simulink model "pruebarc"  (R2025a)
settings: Solver=FixedStepAuto  StartTime=0.0  StopTime=inf  FixedStep=0.001  RelTol=1e-3  EnableMultiTasking=on
model workspace (MAT data in the model file):
  F = [-0.7032  -0.5711  1.7669; 0.2778  -1.4711  1.3647; -0.2558  -0.048  -0.058; -0.11613436  1.15693153  -2.12434445; -0.9531108  1.93997803  -1.59591795; 0.18138056  0.21948418  -0.51411462; 0.946468571296  -1.53366910719  1.49687863641; 1.6173892229  -2.23297604045  1.05599978612; 0.064936415208  -0.401792113254  0.64983001987; -1.4745115325  1.64380224797  -0.507501872867; -2.02779359087  2.31055207818  -0.250825372052; -0.323507655319  0.522799350129  -0.471279686079; 1.62334375322  -1.55174386087  -0.332582390354; 2.13197695059  -2.2289406246  -0.415150203049; 0.493277586385  -0.56171347709  0.16919281873]
  G = [4.2242  -1.1144  -1.3646  0  0  0  0  0  0  0  0  0  0  0  0; -0.011  -5.2505  -0.6752  0  0  0  0  0  0  0  0  0  0  0  0; 0.4464  -0.0899  0.7457  0  0  0  0  0  0  0  0  0  0  0  0; -2.17543118  3.62336232  2.66277077  4.2242  -1.1144  -1.3646  0  0  0  0  0  0  0  0  0; 1.79886694  7.2917437  1.63185763  -0.011  -5.2505  -0.6752  0  0  0  0  0  0  0  0  0; -1.10591356  0.54230172  0.33822368  0.4464  -0.0899  0.7457  0  0  0  0  0  0  0  0  0; -1.45160837282  -5.75407030143  -2.20680687777  -2.17543118  3.62336232  2.66277077  4.2242  -1.1144  -1.3646  0  0  0  0  0  0; -4.75988817257  -8.98023494729  -1.19933418349  1.79886694  7.2917437  1.63185763  -0.011  -5.2505  -0.6752  0  0  0  0  0  0; 0.534272669204  -1.30831327882  -0.779082902646  -1.10591356  0.54230172  0.33822368  0.4464  -0.0899  0.7457  0  0  0  0  0  0; 4.68314952234  6.86321568202  0.860204767951  -1.45160837282  -5.75407030143  -2.20680687777  -2.17543118  3.62336232  2.66277077  4.2242  -1.1144  -1.3646  0  0  0; 7.32813659636  9.82688776962  0.0880751294495  -4.75988817257  -8.98023494729  -1.19933418349  1.79886694  7.2917437  1.63185763  -0.011  -5.2505  -0.6752  0  0  0; 0.568808239237  1.97882463075  0.667256048493  0.534272669204  -1.30831327882  -0.779082902646  -1.10591356  0.54230172  0.33822368  0.4464  -0.0899  0.7457  0  0  0; -6.47326227638  -6.94196363276  0.523779012831  4.68314952234  6.86321568202  0.860204767951  -1.45160837282  -5.75407030143  -2.20680687777  -2.17543118  3.62336232  2.66277077  4.2242  -1.1144  -1.3646; -8.70319020551  -9.84923130785  1.02000189098  7.32813659636  9.82688776962  0.0880751294495  -4.75988817257  -8.98023494729  -1.19933418349  1.79886694  7.2917437  1.63185763  -0.011  -5.2505  -0.6752; -1.58269108232  -2.34207301299  -0.262968836668  0.568808239237  1.97882463075  0.667256048493  0.534272669204  -1.30831327882  -0.779082902646  -1.10591356  0.54230172  0.33822368  0.4464  -0.0899  0.7457]
  H = [22131.1173138 20323.7560581 -1531.64777338 -13284.6672436 -19882.239349 -1189.60000517 7040.1548235 16995.1890063 2962.85657152 -1788.53809124 -12245.5245907 -3182.80208225 ... (225 elements, 15x15)]
  Pc = [-4.2242 0.011 -0.4464 4.2242 -0.011 0.4464 2.17543118 -1.79886694 1.10591356 -2.17543118 1.79886694 -1.10591356 ... (1020 elements, 68x15)]
  Qvec = [50  0  0  0  0  0  0  0  0  0  0  0  0  0  0; 0  50  0  0  0  0  0  0  0  0  0  0  0  0  0; 0  0  50  0  0  0  0  0  0  0  0  0  0  0  0; 0  0  0  50  0  0  0  0  0  0  0  0  0  0  0; 0  0  0  0  50  0  0  0  0  0  0  0  0  0  0; 0  0  0  0  0  50  0  0  0  0  0  0  0  0  0; 0  0  0  0  0  0  50  0  0  0  0  0  0  0  0; 0  0  0  0  0  0  0  50  0  0  0  0  0  0  0; 0  0  0  0  0  0  0  0  50  0  0  0  0  0  0; 0  0  0  0  0  0  0  0  0  50  0  0  0  0  0; 0  0  0  0  0  0  0  0  0  0  50  0  0  0  0; 0  0  0  0  0  0  0  0  0  0  0  50  0  0  0; 0  0  0  0  0  0  0  0  0  0  0  0  122.671454978  -50.1228812954  -14.951064512; 0  0  0  0  0  0  0  0  0  0  0  0  -50.1228812954  218.216126937  -177.895514013; 0  0  0  0  0  0  0  0  0  0  0  0  -14.951064512  -177.895514013  361.167619907]
  Sc = [-0.7032  -0.5711  1.7669; 0.2778  -1.4711  1.3647; -0.2558  -0.048  -0.058; 0.7032  0.5711  -1.7669; -0.2778  1.4711  -1.3647; 0.2558  0.048  0.058; -0.11613436  1.15693153  -2.12434445; -0.9531108  1.93997803  -1.59591795; 0.18138056  0.21948418  -0.51411462; 0.11613436  -1.15693153  2.12434445; 0.9531108  -1.93997803  1.59591795; -0.18138056  -0.21948418  0.51411462; 0.946468571296  -1.53366910719  1.49687863641; 1.6173892229  -2.23297604045  1.05599978612; 0.064936415208  -0.401792113254  0.64983001987; -0.946468571296  1.53366910719  -1.49687863641; -1.6173892229  2.23297604045  -1.05599978612; -0.064936415208  0.401792113254  -0.64983001987; -1.4745115325  1.64380224797  -0.507501872867; -2.02779359087  2.31055207818  -0.250825372052; -0.323507655319  0.522799350129  -0.471279686079; 1.4745115325  -1.64380224797  0.507501872867; 2.02779359087  -2.31055207818  0.250825372052; 0.323507655319  -0.522799350129  0.471279686079; 1.62334375322  -1.55174386087  -0.332582390354; 2.13197695059  -2.2289406246  -0.415150203049; 0.493277586385  -0.56171347709  0.16919281873; -1.62334375322  1.55174386087  0.332582390354; -2.13197695059  2.2289406246  0.415150203049; -0.493277586385  0.56171347709  -0.16919281873; 0  0  0; 0  0  0; 0  0  0; 0  0  0; 0  0  0; 0  0  0; 0  0  0; 0  0  0; 0  0  0; 0  0  0; 0  0  0; 0  0  0; 0  0  0; 0  0  0; 0  0  0; 0  0  0; 0  0  0; 0  0  0; 0  0  0; 0  0  0; 0  0  0; 0  0  0; 0  0  0; 0  0  0; 0  0  0; 0  0  0; 0  0  0; 0  0  0; 0  0  0; 0  0  0; -1.01143611879  0.934917795451  0.497586139165; 1.01143611879  -0.934917795451  -0.497586139165; 1.62334375322  -1.55174386087  -0.332582390354; 2.13197695059  -2.2289406246  -0.415150203049; 0.493277586385  -0.56171347709  0.16919281873; -1.62334375322  1.55174386087  0.332582390354; -2.13197695059  2.2289406246  0.415150203049; -0.493277586385  0.56171347709  -0.16919281873]
  m = 3
  nu = 15
  qc = [1; 1; 0.5; 1; 1; 0.5; 1; 1; 0.5; 1; 1; 0.5; 1; 1; 0.5; 1; 1; 0.5; 1; 1; 0.5; 1; 1; 0.5; 1; 1; 0.5; 1; 1; 0.5; 1.41421356237; 1.41421356237; 2; 1.41421356237; 1.41421356237; 2; 1.41421356237; 1.41421356237; 2; 1.41421356237; 1.41421356237; 2; 1.41421356237; 1.41421356237; 2; 1.41421356237; 1.41421356237; 2; 1.41421356237; 1.41421356237; 2; 1.41421356237; 1.41421356237; 2; 1.41421356237; 1.41421356237; 2; 1.41421356237; 1.41421356237; 2; 1; 1; 1; 1; 0.5; 1; 1; 0.5]
libraries: px4Sensorslib x1
settings Model: SimulationMode=external  ExtModeTrigDuration=10  Creator=The MathWorks, Inc.  LastModifiedBy=aero
settings SolverCC: AlgebraicLoopSolver=TrustRegion  PositivePriorityOrder=on  AutoInsertRateTranBlk=on  MaxZcPerStep=1.0
settings OptimizationCC: EnhancedBackFolding=on  PassReuseOutputArgsAs=Individual arguments  MaxStackSize=64  OptimizeBlockOrder=speed  DifferentSizesBufferReuse=on  OptimizationCustomize=off  EfficientTunableParamExpr=on
settings DebuggingCC: ParameterPrecisionLossMsg=none  ParameterTunabilityLossMsg=error  UnconnectedInputMsg=warning  UnconnectedOutputMsg=warning  UnconnectedLineMsg=warning  SubsystemReferenceDiagnosticForUnitTest=warning  ArithmeticOperatorsInVariantConditions=warning
settings HardwareCC: ProdBitPerPointer=32.0  ProdBitPerSizeT=32.0  ProdBitPerPtrDiffT=32.0  ProdLargestAtomicInteger=Long  ProdLargestAtomicFloat=Double  ProdWordSize=32.0  ProdLongLongMode=on  ProdHWDeviceType=ARM Compatible->ARM Cortex
settings ModelReferenceCC: EnableRefExpFcnMdlSchedulingChecks=on
settings SFSimCC: MATLABDynamicMemAlloc=off  SimTargetLang=C++  SimDLTargetLibrary=mkl-dnn
settings RTWCC: SystemTargetFile=ert.tlc  HardwareBoard=PX4 Pixhawk 6c  TLCOptions="-aInlineSetEventsForThisBaseRateFcn=TLC_FALSE -aSuppressMultiTaskScheduler=TLC_FALSE  -aRateBasedStepFcn=0"  TemplateMakefile=ert_default_tmf  GenerateReport=on  Toolchain=GNU Tools for PX4 Autopilots  IncludeHyperlinkInReport=on  LaunchReport=on  TargetLang=C++  GenerateTraceInfo=on  GenerateTraceReport=on  GenerateTraceReportSl=on  GenerateTraceReportSf=on  GenerateTraceReportEml=on  GPUComputeCapability=3.5  DLArmComputeVersion=19.05  Description=Embedded Coder
settings CodeAppCC: ForceParamTrailComments=on  IgnoreCustomStorageClasses=off  OperatorAnnotations=on  SimulinkDataObjDesc=on  SFDataObjDesc=on  InsertBlockDesc=on
settings ERTTargetCC: ExtModeTransport=3.0  ExtModeStaticAllocSize=1024.0  InlinedParameterPlacement=Hierarchical

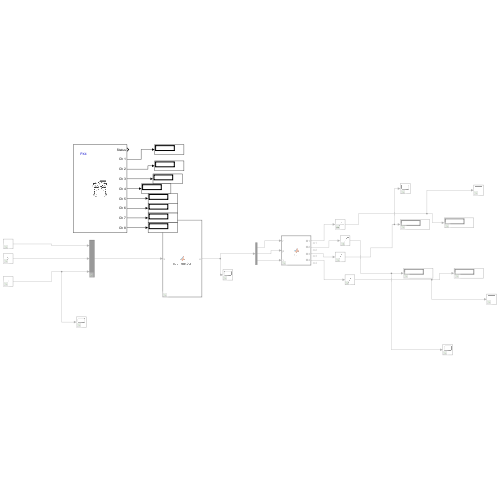
[thumbnail: Simulink's stored preview of the top-level diagram]
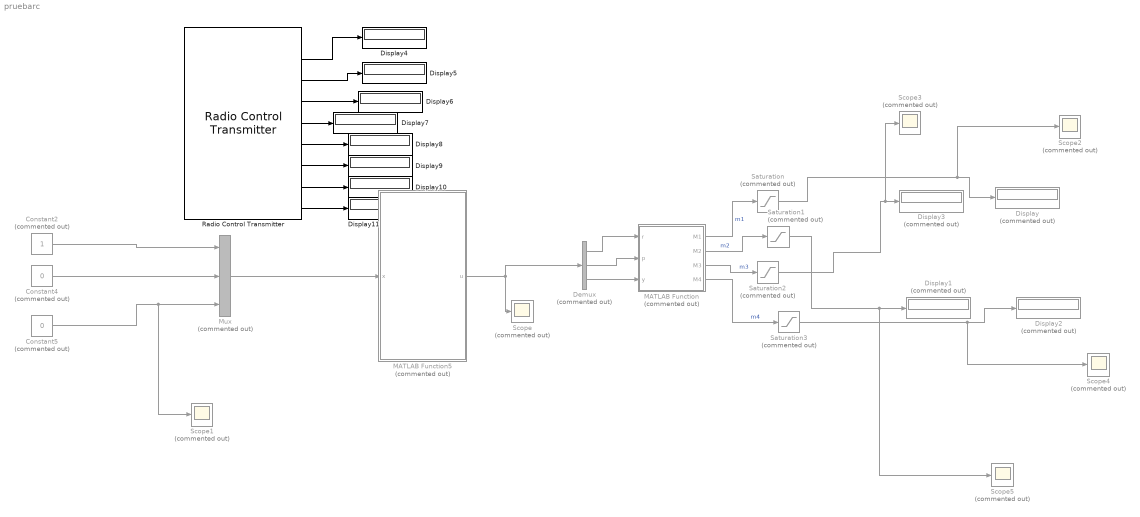
== system pruebarc ==
  Constant2 : Constant  Commented=on
  Constant4 : Constant  Commented=on  Value=0
  Constant5 : Constant  Commented=on  Value=0
  Demux : Demux  Commented=on  Outputs=3
  Display{,1..3} (4 alike) : Display  Commented=on
  Display{4..11} (8 alike) : Display
  MATLAB Function : MATLAB Function  Commented=on  TreatAsAtomicUnit=on  SystemSampleTime=0.0201
  MATLAB Function5 : MATLAB Function  Commented=on  TreatAsAtomicUnit=on  SystemSampleTime=0.0201
  Mux : Mux  Commented=on  Inputs=3
  Radio Control Transmitter : px4Sensorslib/Radio Control Transmitter  channel1=on  channel2=on  channel3=on  channel4=on  channel5=on  channel6=on  channel7=on  channel8=on  channel_count=off  rssi=off  rc_input_source=off  timestamp_last_signal=off  time_stamp=off  sampleTime=1/250  BlockingMode=off  BlockTimeout=5
  Saturation{,1..3} (4 alike) : Saturate  Commented=on  UpperLimit=1  LowerLimit=0
  Scope{,1..5} (6 alike) : Scope  Commented=on
      Scope settings: ActiveDisplayYMinimum=-0.053985449326909025  ActiveDisplayYMaximum=0.097577906132606917
      Scope2 settings: DataLoggingVariableName=ScopeData2
      Scope3 settings: DataLoggingVariableName=ScopeData3
      Scope4 settings: DataLoggingVariableName=ScopeData4
      Scope5 settings: DataLoggingVariableName=ScopeData5
  wires:
  MATLAB Function/2(M2) -> Saturation1/1  "m2"
  Demux/3 -> MATLAB Function/3(y)
  Demux/1 -> MATLAB Function/1(r)
  MATLAB Function5/1(u) -> Demux/1, Scope/1
  MATLAB Function/1(M1) -> Saturation/1  "m1"
  MATLAB Function/4(M4) -> Saturation3/1  "m4"
  Demux/2 -> MATLAB Function/2(p)
  MATLAB Function/3(M3) -> Saturation2/1  "m3"
  Saturation/1 -> Scope2/1, Display/1
  Saturation1/1 -> Scope5/1, Display1/1
  Saturation2/1 -> Scope3/1, Display3/1
  Mux/1 -> MATLAB Function5/1(x)
  Constant5/1 -> Scope1/1, Mux/3
  Constant4/1 -> Mux/2
  Constant2/1 -> Mux/1
  Saturation3/1 -> Scope4/1, Display2/1
  Radio Control Transmitter/2 -> Display4/1
  Radio Control Transmitter/3 -> Display5/1
  Radio Control Transmitter/4 -> Display6/1
  Radio Control Transmitter/5 -> Display7/1
  Radio Control Transmitter/6 -> Display8/1
  Radio Control Transmitter/7 -> Display9/1
  Radio Control Transmitter/8 -> Display10/1
  Radio Control Transmitter/9 -> Display11/1

== matlab function pruebarc/MATLAB Function ==
  data: M1 output; r input; p input; y input; M2 output; M3 output; M4 output
function [M1,M2,M3,M4] = fcn( r, p, y)
% t: thrust
% r: roll
% p: pitch
% y: yaw
persistent trim mixer thrust
% M1 = t + r + p - y;
% M2 = t - r - p - y;
% M3 = t - r + p + y;
% M4 = t + r - p + y;
trim = [0.2691;0.3501;0.2498;0.3462];
thrust = 0.314;
u = [r;p;y; thrust];
mixer = [1 -1 -1 1;
        1 -1 1 -1;
        1 1 -1 -1
        1 1 1 1];
M = mixer\u;
M1= M(1,1)+trim(1,1);
M2= M(2,1)+trim(2,1);
M3= M(3,1)+trim(3,1);
M4= M(4,1)+trim(4,1);

== matlab function pruebarc/MATLAB Function5 ==
  data: x input; u output size=[m 1]; H parameter double; F parameter double; Qvec parameter double; G parameter double; Pc parameter double; qc parameter double; Sc parameter double
function u = mpc_function(x, H, F, Qvec, G, Pc, qc, Sc)
persistent opts x0 u_prev
x = double(x);
if isempty(u_prev)
    u_prev = zeros(3,1,'double');
end

if isempty(x0)
    x0 = zeros(15,1,'double');
end
% uvec = zeros(nu,1);
% === Construcción del QP ===
f = (2*x'*F'*Qvec*G)';

% Resolver QP
if isempty(opts)
opts = optimoptions('quadprog', 'Algorithm','active-set','Display','off');
end
[uvec,a,b] = quadprog(2*H,f, Pc,qc + Sc*x,[],[],[],[],x0, opts);

% Acción de control 
u = zeros(3,1);
if  b > 0
uvec = double(uvec);
u(:) = uvec(1:3);
u_prev = u;
x0= uvec;
else
    u = u_prev;
end
